simulink model "pH_control_loops"  (R2019a)
settings: Solver=VariableStepAuto  StartTime=0.0  StopTime=600  RelTol=1e-3
values from neighbouring files (symbols this model uses):
  pH_const = struct()    [prepare_sim.m]
undefined symbols (not defined in the file or in its folder): sigbuilder_block
settings Model: Creator=User  LastModifiedBy=User
settings DebuggingCC: PregeneratedLibrarySubsystemCodeDiagnostic=none  ArithmeticOperatorsInVariantConditions=warning
settings CodeAppCC: StateflowObjectComments=on

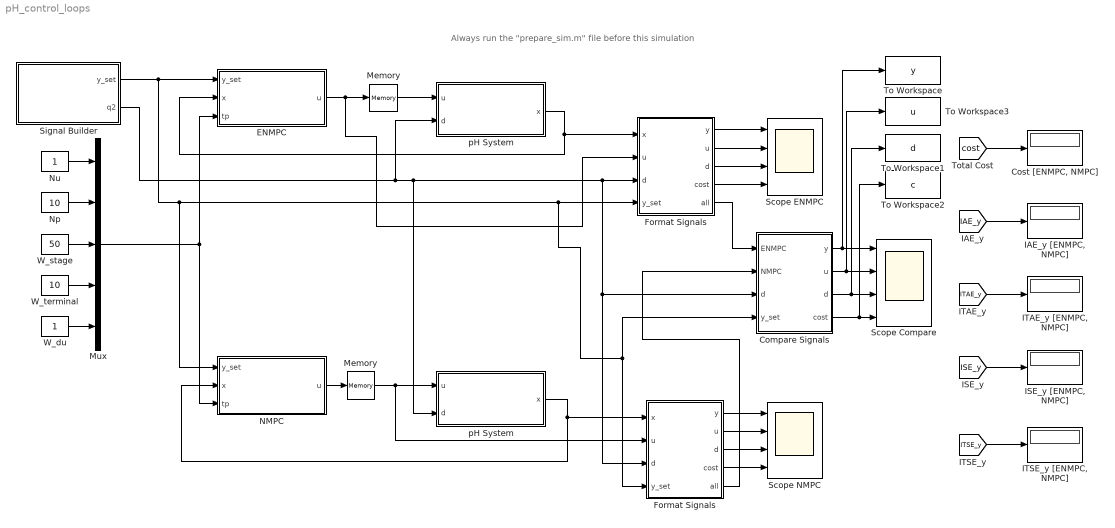
== system pH_control_loops ==
  note: Always run the "prepare_sim.m" file before this simulation
  " Cost [ENMPC, NMPC]" : Display
  " Memory " : Memory  InitialCondition=pH_const.u_0
  " pH System " : Subsystem
  Compare Signals : Subsystem
  ENMPC : Subsystem
  Format Signals : Subsystem
  "Format Signals " : Subsystem
  "IAE_y [ENMPC, NMPC]" : Display
  "ISE_y [ENMPC, NMPC]" : Display
  "ITAE_y [ENMPC, NMPC]" : Display
  "ITSE_y [ENMPC, NMPC]" : Display
  Memory : Memory  InitialCondition=pH_const.u_0
  Mux : Mux  Inputs=5
  NMPC : Subsystem
  Np : Constant  Value=10
  Nu : Constant
  Scope Compare : Scope  NumInputPorts=4
  Scope ENMPC : Scope  NumInputPorts=4
  Scope NMPC : Scope  NumInputPorts=4
  Signal Builder : Subsystem  Tag=STV Subsys  LoadFcn=sigbuilder_block('load');  StartFcn=sigbuilder_block('start');  StopFcn=sigbuilder_block('stop');  ClipboardFcn=sigbuilder_block('clipboard');  mask(Sigbuilder block){tuvar=[0:10]}
      mask help: Simulink:masks:SigbuilderBlock_MD
      mask init:
      | if ~strcmp(get_param(bdroot(gcbh),'SimulationStatus'),'stopped') tuvar = sigbuilder_block('maskInit'); end
      settings: CopyFcn=sigbuilder_block('copy');  DeleteFcn=sigbuilder_block('delete');  ModelCloseFcn=sigbuilder_block('modelClose');  PreSaveFcn=sigbuilder_block('preSave');  PauseFcn=sigbuilder_block('pause');  ContinueFcn=sigbuilder_block('continue');  NameChangeFcn=sigbuilder_block('namechange');  OpenFcn=sigbuilder_block('open',[184.5 249 640.5 331.5 ]);  CloseFcn=sigbuilder_block('close');
      mask Display: plot(0, 0, 100, 100,[2, 2, 32, 32, 2], [68, 8, 8, 68, 68],[32, 2], [38, 38], [32, 19, 2],[53, 60, 44], [32, 17, 17, 2],[16, 16, 31, 31]);txt = getActiveGroup(gcbh);text(2, 100, txt,'verticalAlignment', 'top');
  To Workspace : ToWorkspace  VariableName=y  SaveFormat=Structure With Time  SampleTime=-1
  To Workspace1 : ToWorkspace  VariableName=d  SaveFormat=Structure With Time  SampleTime=-1
  To Workspace2 : ToWorkspace  VariableName=c  SaveFormat=Structure With Time  SampleTime=-1
  To Workspace3 : ToWorkspace  VariableName=u  SaveFormat=Structure With Time  SampleTime=-1
  W_du : Constant
  W_stage : Constant  Value=50
  W_terminal : Constant  Value=10
  pH System : Subsystem
  wires:
  ENMPC/1(u) -> Format Signals/2(" u "), Memory/1
  Signal Builder/1(y_set) -> NMPC/1(y_set), Format Signals/4(y_set), "Format Signals "/4(y_set), Compare Signals/4(y_set), ENMPC/1(y_set)
  pH System/1(x) -> ENMPC/2(x), Format Signals/1(x)
  Nu/1 -> Mux/1
  Np/1 -> Mux/2
  W_stage/1 -> Mux/3
  W_terminal/1 -> Mux/4
  Mux/1 -> ENMPC/3(tp), NMPC/3(tp)
  Format Signals/1(y) -> Scope ENMPC/1
  [IAE_y] -> "IAE_y [ENMPC, NMPC]"/1
  [ITAE_y] -> "ITAE_y [ENMPC, NMPC]"/1
  [ISE_y] -> "ISE_y [ENMPC, NMPC]"/1
  [ITSE_y] -> "ITSE_y [ENMPC, NMPC]"/1
  W_du/1 -> Mux/5
  Format Signals/2(u) -> Scope ENMPC/2
  Format Signals/3(d) -> Scope ENMPC/3
  Format Signals/4(cost) -> Scope ENMPC/4
  [cost] -> " Cost [ENMPC, NMPC]"/1
  Compare Signals/4(cost) -> To Workspace2/1, Scope Compare/4
  Format Signals/5(all) -> Compare Signals/1(ENMPC)
  "Format Signals "/5(all) -> Compare Signals/2(NMPC)
  " Memory "/1 -> " pH System "/1(u), "Format Signals "/2(" u ")
  NMPC/1(u) -> " Memory "/1
  Signal Builder/2(q2) -> " pH System "/2(d), Compare Signals/3(" d "), "Format Signals "/3(" d "), Format Signals/3(" d "), pH System/2(d)
  " pH System "/1(x) -> NMPC/2(x), "Format Signals "/1(x)
  "Format Signals "/1(y) -> Scope NMPC/1
  "Format Signals "/2(u) -> Scope NMPC/2
  "Format Signals "/3(d) -> Scope NMPC/3
  "Format Signals "/4(cost) -> Scope NMPC/4
  Memory/1 -> pH System/1(u)
  Compare Signals/1(y) -> To Workspace/1, Scope Compare/1
  Compare Signals/2(u) -> To Workspace3/1, Scope Compare/2
  Compare Signals/3(d) -> To Workspace1/1, Scope Compare/3

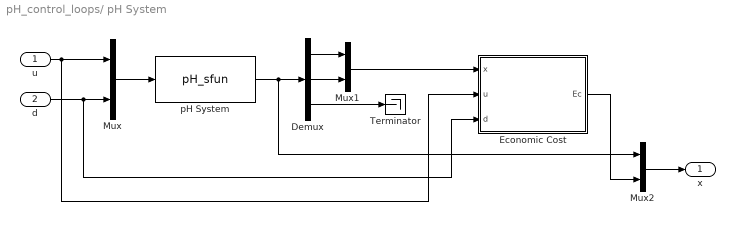
== system pH_control_loops/ pH System  ==
  u : Inport
  d : Inport  Port=2
  Demux : Demux  Outputs=3
  Economic Cost : MATLAB Function  TreatAsAtomicUnit=on
  Mux : Mux  Inputs=2
  Mux1 : Mux  Inputs=2
  Mux2 : Mux  Inputs=2
  Terminator : Terminator
  pH System : S-Function  FunctionName=pH_sfun  SFunctionDeploymentMode=off  EnableBusSupport=off
  x : Outport
  wires:
  d/1 -> Economic Cost/3(d), Mux/2
  Mux/1 -> pH System/1
  u/1 -> Mux/1, Economic Cost/2(u)
  pH System/1 -> Mux2/1, Demux/1
  Mux1/1 -> Economic Cost/1(x)
  Mux2/1 -> x/1
  Demux/1 -> Mux1/1
  Demux/2 -> Mux1/2
  Demux/3 -> Terminator/1
  Economic Cost/1(Ec) -> Mux2/2

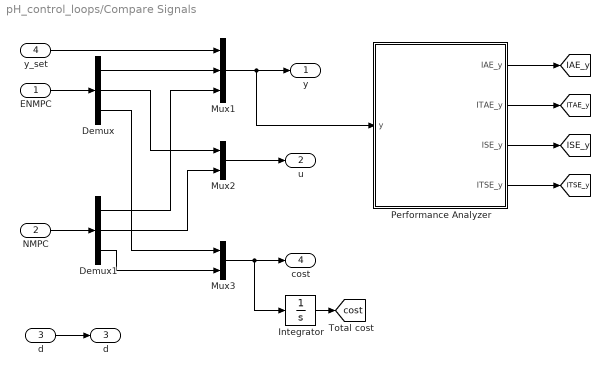
== system pH_control_loops/Compare Signals ==
  ENMPC : Inport
  NMPC : Inport  Port=2
  " d " : Inport  Port=3
  y_set : Inport  Port=4
  Demux : Demux  Outputs=3
  Demux1 : Demux  Outputs=3
  Integrator : Integrator
  Mux1 : Mux  Inputs=3
  Mux2 : Mux  Inputs=2
  Mux3 : Mux  Inputs=2
  Performance Analyzer : Subsystem
  y : Outport
  u : Outport  Port=2
  d : Outport  Port=3
  cost : Outport  Port=4
  tag scope: IAE_y=global, ISE_y=global, ITAE_y=global, ITSE_y=global, cost=global
  wires:
  ENMPC/1 -> Demux/1
  Performance Analyzer/1(IAE_y) -> [IAE_y]
  Performance Analyzer/3(ISE_y) -> [ISE_y]
  Performance Analyzer/2(ITAE_y) -> [ITAE_y]
  Performance Analyzer/4(ITSE_y) -> [ITSE_y]
  Demux/2 -> Mux2/1
  Demux/1 -> Mux1/2
  y_set/1 -> Mux1/1
  Demux1/1 -> Mux1/3
  Demux1/2 -> Mux2/2
  NMPC/1 -> Demux1/1
  Mux1/1 -> Performance Analyzer/1(y), y/1
  " d "/1 -> d/1
  Demux/3 -> Mux3/1
  Demux1/3 -> Mux3/2
  Mux2/1 -> u/1
  Mux3/1 -> Integrator/1, cost/1
  Integrator/1 -> [cost]

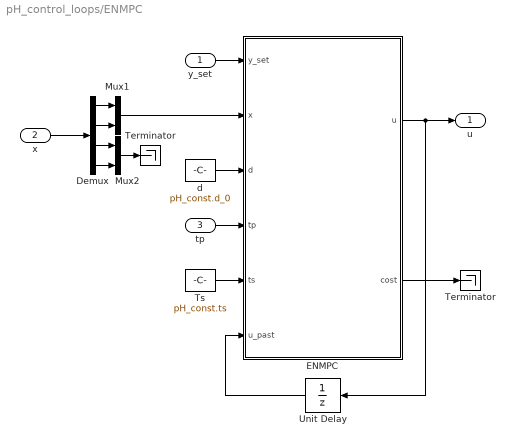
== system pH_control_loops/ENMPC ==
  y_set : Inport
  x : Inport  Port=2
  tp : Inport  Port=3
  Demux : Demux
  "ENMPC " : MATLAB Function  TreatAsAtomicUnit=on  SystemSampleTime=pH_const.ts
  Mux1 : Mux  Inputs=2
  Mux2 : Mux  Inputs=2
  Terminator : Terminator
  "Terminator " : Terminator
  Ts : Constant  Value=pH_const.ts
  Unit Delay : UnitDelay  InitialCondition=pH_const.u_0  SampleTime=pH_const.ts  HasFrameUpgradeWarning=on
  d : Constant  Value=pH_const.d_0
  u : Outport
  wires:
  "ENMPC "/1(u) -> Unit Delay/1, u/1
  Unit Delay/1 -> "ENMPC "/6(u_past)
  y_set/1 -> "ENMPC "/1(y_set)
  x/1 -> Demux/1
  tp/1 -> "ENMPC "/4(tp)
  d/1 -> "ENMPC "/3(d)
  Ts/1 -> "ENMPC "/5(ts)
  "ENMPC "/2(cost) -> "Terminator "/1
  Demux/1 -> Mux1/1
  Demux/2 -> Mux1/2
  Mux1/1 -> "ENMPC "/2(x)
  Demux/4 -> Mux2/2
  Demux/3 -> Mux2/1
  Mux2/1 -> Terminator/1

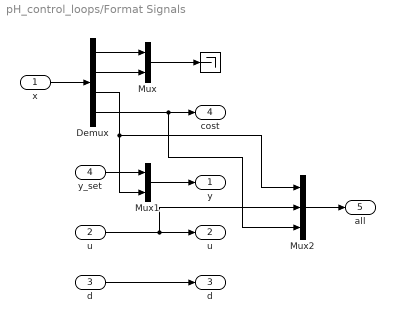
== system pH_control_loops/Format Signals ==
  x : Inport
  " u " : Inport  Port=2
  " d " : Inport  Port=3
  y_set : Inport  Port=4
  "  " : Terminator
  Demux : Demux
  Mux : Mux  Inputs=2
  Mux1 : Mux  Inputs=2
  Mux2 : Mux  Inputs=3
  y : Outport
  u : Outport  Port=2
  d : Outport  Port=3
  cost : Outport  Port=4
  all : Outport  Port=5
  wires:
  x/1 -> Demux/1
  Demux/3 -> Mux1/2, Mux2/1
  Demux/2 -> Mux/2
  Demux/1 -> Mux/1
  Mux/1 -> "  "/1
  y_set/1 -> Mux1/1
  " u "/1 -> Mux2/2, u/1
  Mux1/1 -> y/1
  " d "/1 -> d/1
  Mux2/1 -> all/1
  Demux/4 -> Mux2/3, cost/1

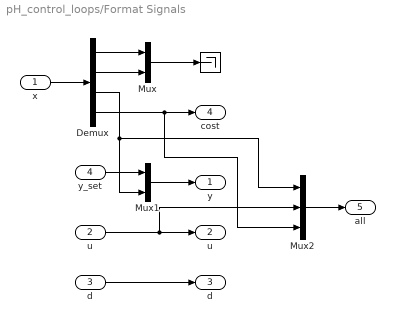
== system pH_control_loops/Format Signals  ==
  x : Inport
  " u " : Inport  Port=2
  " d " : Inport  Port=3
  y_set : Inport  Port=4
  "  " : Terminator
  Demux : Demux
  Mux : Mux  Inputs=2
  Mux1 : Mux  Inputs=2
  Mux2 : Mux  Inputs=3
  y : Outport
  u : Outport  Port=2
  d : Outport  Port=3
  cost : Outport  Port=4
  all : Outport  Port=5
  wires:
  x/1 -> Demux/1
  Demux/3 -> Mux1/2, Mux2/1
  Demux/2 -> Mux/2
  Demux/1 -> Mux/1
  Mux/1 -> "  "/1
  y_set/1 -> Mux1/1
  " u "/1 -> Mux2/2, u/1
  Mux1/1 -> y/1
  " d "/1 -> d/1
  Mux2/1 -> all/1
  Demux/4 -> cost/1, Mux2/3

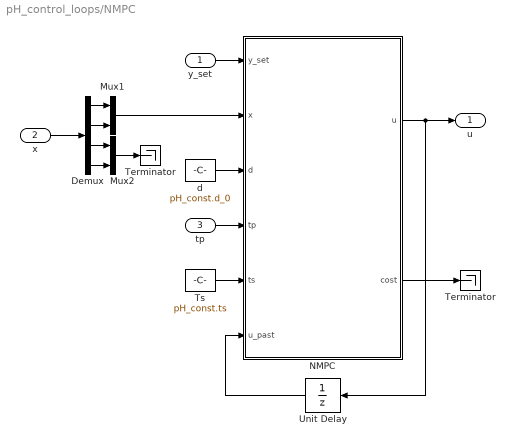
== system pH_control_loops/NMPC ==
  y_set : Inport
  x : Inport  Port=2
  tp : Inport  Port=3
  Demux : Demux
  Mux1 : Mux  Inputs=2
  Mux2 : Mux  Inputs=2
  "NMPC " : MATLAB Function  TreatAsAtomicUnit=on  SystemSampleTime=pH_const.ts
  Terminator : Terminator
  "Terminator " : Terminator
  Ts : Constant  Value=pH_const.ts
  Unit Delay : UnitDelay  InitialCondition=pH_const.u_0  SampleTime=pH_const.ts  HasFrameUpgradeWarning=on
  d : Constant  Value=pH_const.d_0
  u : Outport
  wires:
  "NMPC "/1(u) -> Unit Delay/1, u/1
  Unit Delay/1 -> "NMPC "/6(u_past)
  y_set/1 -> "NMPC "/1(y_set)
  tp/1 -> "NMPC "/4(tp)
  d/1 -> "NMPC "/3(d)
  Ts/1 -> "NMPC "/5(ts)
  "NMPC "/2(cost) -> Terminator/1
  x/1 -> Demux/1
  Mux2/1 -> "Terminator "/1
  Mux1/1 -> "NMPC "/2(x)
  Demux/4 -> Mux2/2
  Demux/2 -> Mux1/2
  Demux/1 -> Mux1/1
  Demux/3 -> Mux2/1

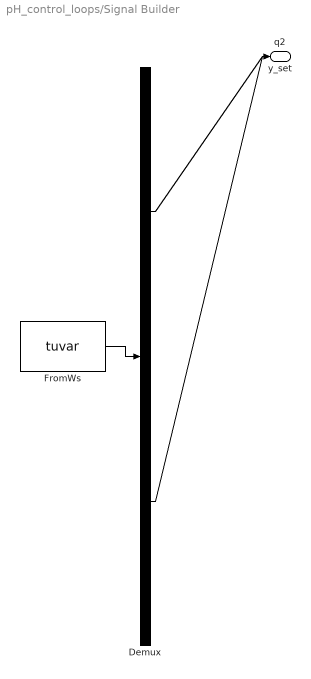
== system pH_control_loops/Signal Builder ==
  Demux : Demux  Tag=STV Demux  Outputs=2
  FromWs : FromWorkspace  Tag=STV FromWs  VariableName=tuvar  SampleTime=0
      SigBuilderData=|
      | common.afterFinalStr = 'Extrapolate'
      | common.sampleTime = 0
      | dataSet(1).timeRange = [0 600]
      | dataSet(1).name = 'Servo'
      | dataSet(2).timeRange = [0 600]
      | dataSet(2).name = 'Regulatory'
      | sbobj.Groups(1).Name = 'Servo'
      | sbobj.Groups(1).Signals(1).Name = 'y_set'
      | sbobj.Groups(1).Signals(1).XData = [0 150 150 300 300 450 450 600]
      | sbobj.Groups(1).Signals(1).YData = [9 9 4 4 7 7 10 10]
      | sbobj.Groups(1).Signals(2).Name = 'q2'
      | sbobj.Groups(1).Signals(2).XData = [0 600]
      | sbobj.Groups(1).Signals(2).YData = [0.55 0.55]
      | sbobj.Groups(1).TimeRange = [0 600]
      | sbobj.Groups(2).Name = 'Regulatory'
      | sbobj.Groups(2).Signals(1).Name = 'y_set'
      | sbobj.Groups(2).Signals(1).XData = [0 600]
      | sbobj.Groups(2).Signals(1).YData = [7 7]
      | sbobj.Groups(2).Signals(2).Name = 'q2'
      | sbobj.Groups(2).Signals(2).XData = [0 150 150 300 300 450 450 600]
      | sbobj.Groups(2).Signals(2).YData = [1.5 1.5 0.25 0.25 2 2 0.55 0.55]
      | sbobj.Groups(2).TimeRange = [0 600]
  y_set : Outport  Tag=STV Outport
  q2 : Outport  Tag=STV Outport  Port=2
  wires:
  FromWs/1 -> Demux/1
  Demux/1 -> y_set/1
  Demux/2 -> q2/1

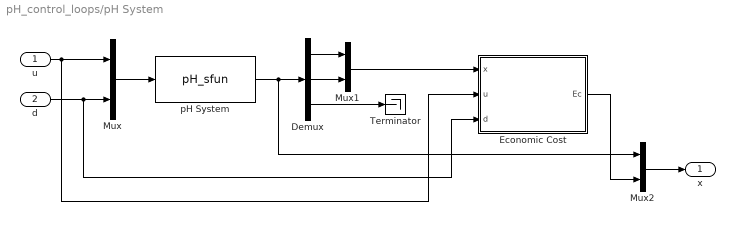
== system pH_control_loops/pH System ==
  u : Inport
  d : Inport  Port=2
  Demux : Demux  Outputs=3
  Economic Cost : MATLAB Function  TreatAsAtomicUnit=on
  Mux : Mux  Inputs=2
  Mux1 : Mux  Inputs=2
  Mux2 : Mux  Inputs=2
  Terminator : Terminator
  pH System : S-Function  FunctionName=pH_sfun  SFunctionDeploymentMode=off  EnableBusSupport=off
  x : Outport
  wires:
  u/1 -> Mux/1, Economic Cost/2(u)
  d/1 -> Economic Cost/3(d), Mux/2
  Mux/1 -> pH System/1
  pH System/1 -> Mux2/1, Demux/1
  Demux/2 -> Mux1/2
  Demux/1 -> Mux1/1
  Mux1/1 -> Economic Cost/1(x)
  Economic Cost/1(Ec) -> Mux2/2
  Demux/3 -> Terminator/1
  Mux2/1 -> x/1

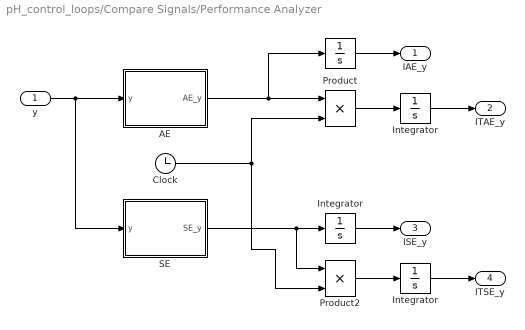
== system pH_control_loops/Compare Signals/Performance Analyzer ==
  y : Inport
  "   " : Integrator
  "    Integrator    " : Integrator
  "   Integrator " : Integrator
  "   Integrator  " : Integrator
  AE : MATLAB Function  TreatAsAtomicUnit=on  SystemSampleTime=pH_const.ts
  Clock : Clock
  Product : Product
  Product2 : Product
  SE : MATLAB Function  TreatAsAtomicUnit=on  SystemSampleTime=pH_const.ts
  IAE_y : Outport
  ITAE_y : Outport  Port=2
  ISE_y : Outport  Port=3
  ITSE_y : Outport  Port=4
  wires:
  y/1 -> SE/1(y), AE/1(y)
  AE/1(AE_y) -> "   "/1, Product/1
  Product/1 -> "   Integrator "/1
  "   Integrator "/1 -> ITAE_y/1
  "   "/1 -> IAE_y/1
  SE/1(SE_y) -> Product2/1, "    Integrator    "/1
  Clock/1 -> Product2/2, Product/2
  Product2/1 -> "   Integrator  "/1
  "    Integrator    "/1 -> ISE_y/1
  "   Integrator  "/1 -> ITSE_y/1

== matlab function pH_control_loops/Compare Signals/Performance Analyzer/AE ==
  data: y input; AE_y output
function AE_y = AE(y)
    y_set = y(1);
    y_ENMPC = y(2);
    y_NMPC = y(3);
    AE_y = [abs(y_ENMPC - y_set);abs(y_NMPC - y_set)];
end

== matlab function pH_control_loops/ENMPC/ENMPC  ==
  data: u output size=[1,1]; cost output size=[1,1]; y_set input; x input; d input; tp input; ts input; u_past input
function [u, cost] = enmpc(y_set,x,d,tp,ts,u_past)
    u = u_past; cost = 0;
    coder.extrinsic('get_control_input');
    [u,cost] = get_control_input(y_set,x,u_past,d,tp,1,ts);
end

== matlab function pH_control_loops/Compare Signals/Performance Analyzer/SE ==
  data: y input; SE_y output
function SE_y = SE(y)
    y_set = y(1);
    y_ENMPC = y(2);
    y_NMPC = y(3);
    SE_y = [(y_ENMPC - y_set)^2;(y_NMPC - y_set)^2];
end

== matlab function pH_control_loops/NMPC/NMPC  ==
  data: u output size=[1,1]; cost output size=[1,1]; y_set input; x input; d input; tp input; ts input; u_past input
function [u, cost] = nmpc(y_set,x,d,tp,ts,u_past)
    u = u_past; cost = 0;
    coder.extrinsic('get_control_input');
    [u,cost] = get_control_input(y_set,x,u_past,d,tp,2,ts);
end

== matlab function pH_control_loops/pH System/Economic Cost ==
  data: x input; u input; Ec output; d input
function Ec = cost(x,u,d)
    Ec = 0;
    coder.extrinsic('ode_set');
    [~,~,Ec] = ode_set(x,u,d);
end

== matlab function pH_control_loops/ pH System /Economic Cost ==
  data: x input; u input; Ec output; d input
function Ec = cost(x,u,d)
    Ec = 0;
    coder.extrinsic('ode_set');
    [~,~,Ec] = ode_set(x,u,d);
end
